simulink model "diff_eq"  (R2020a)
settings: Solver=VariableStepAuto  StartTime=0.0  StopTime=10.0  RelTol=1e-3
settings Model: Creator=u_deliz  LastModifiedBy=u_deliz

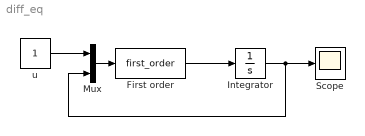
== system diff_eq ==
  First order : MATLABFcn  MATLABFcn=first_order  OutputDimensions=2
  Integrator : Integrator  InitialCondition=0.5
  Mux : Mux  Inputs=2
  Scope : Scope
  u : Constant
  wires:
  First order/1 -> Integrator/1
  Integrator/1 -> Mux/2, Scope/1
  u/1 -> Mux/1
  Mux/1 -> First order/1
